simulink model "mirageTracking"  (Simulink 8.5)
settings: Solver=FixedStepDiscrete  StartTime=0.0  StopTime=1  FixedStep=0.1  RelTol=1e-3
undefined symbols (not defined in the file or in its folder): IsPositionTracked, IsSkeletonTracked, JointDepthIndices, JointImageIndices, JointTrackingState, JointWorldCoordinates, none, PositionDepthIndices, PositionImageIndices, PositionWorldCoordinates, SegmentationData, SkeletonTrackingID, videoinput
libraries: imaqlib x2
settings Model: Creator=sd0016  LastModifiedBy=sd0016  CovSFcnEnable=off
settings DataIOCC: SignalLoggingSaveFormat=Dataset
settings OptimizationCC: ExpressionDepthLimit=128
settings DebuggingCC: UnderspecifiedInitializationDetection=Simplified  MergeDetectMultiDrivingBlocksExec=error  SolverPrmCheckMsg=warning  FcnCallInpInsideContextMsg=EnableAllAsError  StateNameClashWarn=none
settings GRTTargetCC: CombineOutputUpdateFcns=on  GRTInterface=off

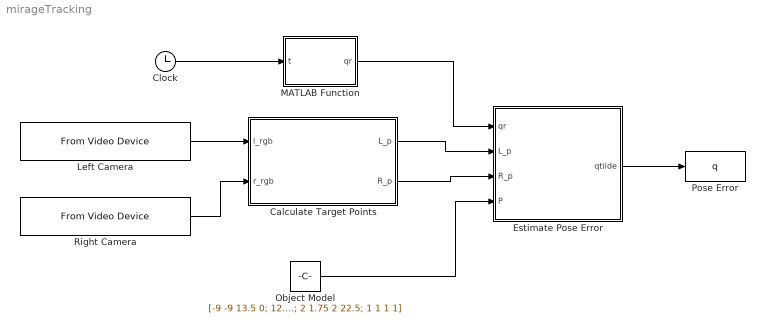
== system mirageTracking ==
  Calculate Target Points : MATLAB Function  TreatAsAtomicUnit=on
  Clock : Clock
  Estimate Pose Error : MATLAB Function  TreatAsAtomicUnit=on
  Left Camera : imaqlib/From Video Device  DeviceMenu=winvideo 1 (Logitech HD Webcam C525)  Device=winvideo 1 (Logitech HD Webcam C525)  ObjConstructor=videoinput('winvideo', 1)  VideoFormatMenu=RGB24_1280x960  VideoFormat=RGB24_1280x960  VideoSource=input1  ROIPosition=[0 0 960 1280]  EnableHWTrigger=off  TriggerConfiguration=none/none  SampleTime=0.1  OutputPortsMode=One multidimensional signal  DataType=single  CanDoHWTrigger=no  ReturnedColorSpace=rgb  BlockHandle=1921.0006  ROIWidth=1280  ROIHeight=960  ROIColumn=0  ROIRow=0  EngXMLPath=C:\Program Files\MATLAB\R2015a\toolbox\imaq\imaq\private  DevXMLPath=C:\MATLAB\SupportPackages\R2015a\osgenericvideointerface\toolbox\imaq\supportpackages\genericvideo\adaptor\win64  EngLibPath=C:\Program Files\MATLAB\R2015a\toolbox\imaq\imaqblks\imaqmex\win64  ColorSpace=rgb  BayerSensorAlignment=grbg  AllMetadata=IsPositionTracked;IsSkeletonTracked;JointDepthIndices;JointImageIndices;JointTrackingState;JointWorldCoordinates;PositionDepthIndices;PositionImageIndices;PositionWorldCoordinates;SegmentationData;SkeletonTrackingID
  MATLAB Function : MATLAB Function  TreatAsAtomicUnit=on
  Object Model : Constant  Value=[-9 -9 13.5 0; 12.75 -12.75 0 0; 2 1.75 2 22.5; 1 1 1 1]  VectorParams1D=off
  Pose Error : ToWorkspace  VariableName=q  SampleTime=-1
  Right Camera : imaqlib/From Video Device  DeviceMenu=winvideo 2 (Logitech HD Webcam C525)  Device=winvideo 2 (Logitech HD Webcam C525)  ObjConstructor=videoinput('winvideo', 2)  VideoFormatMenu=RGB24_1280x960  VideoFormat=RGB24_1280x960  VideoSource=input1  ROIPosition=[0 0 960 1280]  EnableHWTrigger=off  TriggerConfiguration=none/none  SampleTime=0.1  OutputPortsMode=One multidimensional signal  DataType=single  CanDoHWTrigger=no  ReturnedColorSpace=rgb  BlockHandle=1921.0006  ROIWidth=1280  ROIHeight=960  ROIColumn=0  ROIRow=0  EngXMLPath=C:\Program Files\MATLAB\R2015a\toolbox\imaq\imaq\private  DevXMLPath=C:\MATLAB\SupportPackages\R2015a\osgenericvideointerface\toolbox\imaq\supportpackages\genericvideo\adaptor\win64  EngLibPath=C:\Program Files\MATLAB\R2015a\toolbox\imaq\imaqblks\imaqmex\win64  ColorSpace=rgb  BayerSensorAlignment=grbg  AllMetadata=IsPositionTracked;IsSkeletonTracked;JointDepthIndices;JointImageIndices;JointTrackingState;JointWorldCoordinates;PositionDepthIndices;PositionImageIndices;PositionWorldCoordinates;SegmentationData;SkeletonTrackingID
  wires:
  Clock/1 -> MATLAB Function/1(t)
  Left Camera/1 -> Calculate Target Points/1(l_rgb)
  Right Camera/1 -> Calculate Target Points/2(r_rgb)
  MATLAB Function/1(qr) -> Estimate Pose Error/1(qr)
  Calculate Target Points/1(L_p) -> Estimate Pose Error/2(L_p)
  Calculate Target Points/2(R_p) -> Estimate Pose Error/3(R_p)
  Object Model/1 -> Estimate Pose Error/4(P)
  Estimate Pose Error/1(qtilde) -> Pose Error/1

== matlab function Calculate Target Points ==
  data: l_rgb input double; L_p output double; r_rgb input double; R_p output double
function [L_p, R_p] = getCenter(l_rgb,r_rgb)

    %#codegen
    L_p=zeros(2,4);
    R_p=zeros(2,4);
    
    %input left image(l_rgb), right image(r_rgb), Pose target position 
    [m,n,c]=size(l_rgb);
    
    %define image variables for processing
    l_gray=zeros(m,n);      r_gray=zeros(m,n);
    l_rgb1=zeros(m,n,c);    r_rgb1=zeros(m,n,c);
    l_rgb2=zeros(m,n);      r_rgb2=zeros(m,n);

    l_bw=false(m,n);        r_bw=false(m,n);

    l_rgb1 = imcomplement(l_rgb);        % converts RGB to CMY color space 
    r_rgb1 = imcomplement(r_rgb);        % converts RGB to CMY color space 
    
    l_gray = 0.2989 * l_rgb1(:,:,1) + 0.5870 * l_rgb1(:,:,2) + 0.1140 * l_rgb1(:,:,3); % rgb2gray(rgb) ;convert rgb to grayscale 
    r_gray = 0.2989 * r_rgb1(:,:,1) + 0.5870 * r_rgb1(:,:,2) + 0.1140 * r_rgb1(:,:,3); % rgb2gray(rgb) ;convert rgb to grayscale
    
    l_rgb2 = l_rgb1(:,:,3)-l_gray;       % imsubtract(rgb1(:,:,3),gray)
    r_rgb2 = r_rgb1(:,:,3)-r_gray;       % imsubtract(rgb1(:,:,3),gray) 
    
    l_rgb2 = medfilt2(l_rgb2);     % medfilt2(rgb2,[3 3]);
    r_rgb2 = medfilt2(r_rgb2);     % medfilt2(rgb2,[3 3]);
    
    l_rgb2 = myMat2gray(l_rgb2);
    r_rgb2 = myMat2gray(r_rgb2);
    
    l_bw = l_rgb2 > 0.6;
    r_bw = r_rgb2 > 0.6;

    %finds yellow regions in image using BlobAnalysis.
    hblob = vision.BlobAnalysis;

    [~,l_center,~] = step(hblob, l_bw); % get [x y] is a centroid of region
    [~,r_center,~] = step(hblob, r_bw); % get [x y] is a centroid of region
    
    %Send Left Camera Points
    ml = size(l_center,1);
    if ml > 4
        ml = 4;
    end
    for i=1:ml
        L_p(:,i)=l_center(i,:);
    end
    
    %Send Right Camera Points
    mr = size(r_center,1);
    if mr > 4
        mr = 4;
    end
    for i=1:mr
        R_p(:,i)=r_center(i,:);
    end
    
    L_p = orderPoints(L_p); 
    R_p = orderPoints(R_p);
    
    
    coder.extrinsic('imshow','plot');
    imshow(l_rgb2);hold on;
    plot(L_p(1,:),L_p(2,:),'ro');
    
    L_p(2,:) = m - L_p(2,:);
    R_p(2,:) = m - R_p(2,:);
end

function imgOut = myMat2gray(imgIn)
    %#codegen
    imgIn = double(imgIn);
    
    minL = min(imgIn(:));
    
    imgTmp = (imgIn - minL);
    
    maxL = max(imgTmp(:));
    
    imgOut = imgTmp/maxL;
end

== matlab function MATLAB Function ==
  data: t input double; qr output double
function qr  = desired(t)
%#codegen

% qr = [xr yr thetar]^T (reference trajectory)
% ur = [vr omegar]^T (reference control input that generates the reference trajetory in ideal conditions)

% A = 1;
% xL = 10;
% vx = 1;

% % 
% % desired x and y 
% xr = vx*t;
% yr = A*sin(2*pi*xr/xL);
% 
% % desired x and y derivatives
% xrdot = vx;
% yrdot = A*(2*pi/xL)*cos(2*pi*xr/xL);
% 
% % desired theta
% thetar = atan2(yrdot,xrdot);
% 
% % desired second derivatives
% xrddot = 0;
% yrddot = -A*(2*pi/xL)^2*sin(2*pi*xr/xL);
% 
% % desired theta derivative
% thetardot = (yrddot - xrddot*tan(thetar))/(xrdot*(1+tan(thetar)^2));
% 
% 
% vr     = sqrt(xrdot^2+yrdot^2);
% omegar = thetardot;

%--------------------------------------------
% 
% xr = vx*t - 30;
% yr = A*sin(2*pi*xr/xL) + 2;
% 
% % desired x and y derivatives
% xrdot = vx;
% yrdot = A*(2*pi/xL)*cos(2*pi*xr/xL);
% 
% % desired theta
% thetar = atan2(yrdot,xrdot);
% 
% % desired second derivatives
% xrddot = 0;
% yrddot = -A*(2*pi/xL)^2*sin(2*pi*xr/xL);
% 
% % desired theta derivative
% thetardot = (yrddot - xrddot*tan(thetar))/(xrdot*(1+tan(thetar)^2));
% 
% vr     = sqrt(xrdot^2+yrdot^2);
% omegar = thetardot;

%--------------------------------------------
% yr = vx*t - 30;
% xr = A*sin(2*pi*yr/xL) + 2;
% 
% yrdot = vx;
% xrdot = A*(2*pi/xL)*cos(2*pi*xr/xL);
% 
% desired theta
% thetar = atan2(yrdot,xrdot);
% thetardot = 0;
% 
% vr     = sqrt(xrdot^2+yrdot^2);
% omegar = thetardot;

%--------------------------------------------
% xr = vx*t - 30;
% yr = 5;
% 
% xrdot = vx;
% yrdot = 0;
% 
% thetar = 0;
% thetardot = 0;
% 
% vr     = sqrt(xrdot^2+yrdot^2);
% omegar = thetardot;

% qr = [xr;yr;thetar];
% ur = [vr;omegar];

qr = [-395 2 45 0 0 0]';

== matlab function Estimate Pose Error ==
  data: qr input double; qtilde output double; L_p input double; R_p input double; P input double
function qtilde = mirage(qr,L_p,R_p,P)
%#codegen

%Desired Robot Pose for current step qr()
robotPoseDes.x = qr(1);
robotPoseDes.y = qr(2);
robotPoseDes.z = qr(3);
robotPoseDes.phi = qr(4);
robotPoseDes.theta = qr(5);
robotPoseDes.psi = qr(6);

%Transform target points from I space into Desired Robot Space
world2robotDes = inv(EulerTrans(robotPoseDes));
S_PDes = world2robotDes*P;

%Calculate the error parameters for current step
errParams = visioMotor(L_p,R_p,S_PDes);

poseErrorMat = eye(4,4);
poseErrorMat(1:3,:) = reshape(errParams,3,4);

world2robot = poseErrorMat*world2robotDes;

robotPoseEst = calculatePose(world2robot);

qtilde = [ -robotPoseEst.x  - robotPoseDes.x;
           -robotPoseEst.y  - robotPoseDes.y;
           -robotPoseEst.z  - robotPoseDes.z;
           -robotPoseEst.phi  - robotPoseDes.phi;
           -robotPoseEst.theta  - robotPoseDes.theta;
           -robotPoseEst.psi  - robotPoseDes.psi;];
       
end
